simulink model "Sandbox"  (R2023a)
settings: Solver=FixedStepAuto  StartTime=0.0  StopTime=10  FixedStep=0.0001  RelTol=1e-3
values from neighbouring files (symbols this model uses):
  AEP = 0.03    [simulation_setup.m]
  PEP = -0.03    [simulation_setup.m]
  step_height = 0.06    [InitialisationScript.m]    (also in simulation_setup.m)
settings Model: Creator=basti  LastModifiedBy=basti
settings SolverCC: ZeroCrossControl=EnableAll  EnableFixedStepZeroCrossing=on
settings ExplorerConfigSet: InternalSimMechanicsExplorerSettings="<ExplorerConfiguration><canonicalview>planar_xy</canonicalview><AnimationSetting><BasePlaybackSpeed>1.0</BasePlaybackSpeed><PlaybackSpeedFactor>1.0</PlaybackSpeedFactor></AnimationSetting><TilePanel><TileInfo><Tiles Columns=\"1\" Count=\"1\" Rows=\"1\"><Column Weight=\"1\"/><Row Weight=\"1\"/><Tile Height=\"1\" Width=\"1\" X=\"0\" Y=\"0\"/></Tiles></TileInfo><SceneInfo><SceneViewer><BGColor><R>0.800000011920928955</R><G>0.800000011920928955</G><B>0.800000011920928955</B></BGColor><Camera><DoPerspective>off</DoPerspective><Position><X>166.088793964076217</X><Y>-65.4585895917369385</Y><Z>6.56230393982627103</Z></Position><Center><X>0.420963900477701602</X><Y>-0.147668832830340768</Y><Z>0.227388390891763464</Z></Center><Up><X>-0.0260738065319616186</X><Y>0.030778444548253292</Y><Z>0.999186090757934631</Z></Up><ViewLimDist>1</ViewLimDist><YLim>0.165421804575422993</YLim><XLim>0.319699403368922774</XLim></Camera></SceneViewer></SceneInfo></TilePanel><MechEditorPanel><Cameras/><GfxPanelCameraMap/><VideoCreator><PlaybackSpeedRatio>1.0</PlaybackSpeedRatio><FrameRate>30</FrameRate><VideoFormat>Motion JPEG AVI</VideoFormat><FrameSize>auto</FrameSize></VideoCreator></MechEditorPanel></ExplorerConfiguration>"

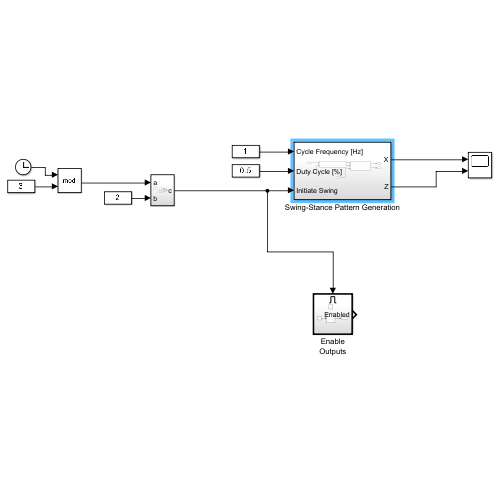
[thumbnail: Simulink's stored preview of the top-level diagram]
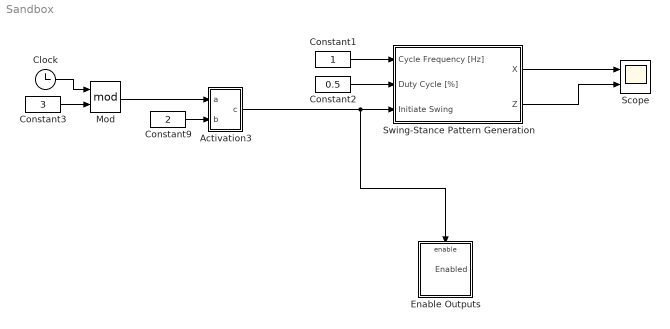
== system Sandbox ==
  Activation3 : Subsystem
  Clock : Clock
  Constant1 : Constant
  Constant2 : Constant  Value=0.5
  Constant3 : Constant  Value=3
  Constant9 : Constant  Value=2
  Enable Outputs : Subsystem  TreatAsAtomicUnit=on
  Mod : Math  Operator=mod
  Scope : Scope  NumInputPorts=2
  Swing-Stance Pattern Generation : Subsystem
  wires:
  Constant9/1 -> Activation3/2(b)
  Swing-Stance Pattern Generation/1(X) -> Scope/1
  Swing-Stance Pattern Generation/2(Z) -> Scope/2
  Activation3/1(c) -> Swing-Stance Pattern Generation/3(Initiate Swing), Enable Outputs/Enable
  Constant2/1 -> Swing-Stance Pattern Generation/2(Duty Cycle [%])
  Constant1/1 -> Swing-Stance Pattern Generation/1(Cycle Frequency [Hz])
  Clock/1 -> Mod/1
  Mod/1 -> Activation3/1(a)
  Constant3/1 -> Mod/2

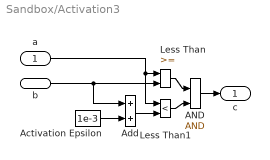
== system Sandbox/Activation3 ==
  a : Inport
  b : Inport  Port=2
  AND : Logic  IconShape=distinctive  AllPortsSameDT=off  OutDataTypeStr=boolean
  Activation Epsilon : Constant  Value=1e-3
  Add : Sum
  Less Than : RelationalOperator  OutDataTypeStr=boolean  RndMeth=Simplest  InputSameDT=off
  Less Than1 : RelationalOperator  Operator=<  OutDataTypeStr=boolean  RndMeth=Simplest  InputSameDT=off
  c : Outport
  wires:
  a/1 -> Less Than1/1, Less Than/1
  Less Than/1 -> AND/1
  Less Than1/1 -> AND/2
  Add/1 -> Less Than1/2
  b/1 -> Add/1, Less Than/2
  AND/1 -> c/1
  Activation Epsilon/1 -> Add/2

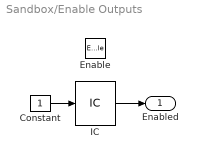
== system Sandbox/Enable Outputs ==
  Enable : EnablePort
  Constant : Constant
  IC : InitialCondition  Value=0
  Enabled : Outport  InitialOutput=0
  wires:
  Constant/1 -> IC/1
  IC/1 -> Enabled/1

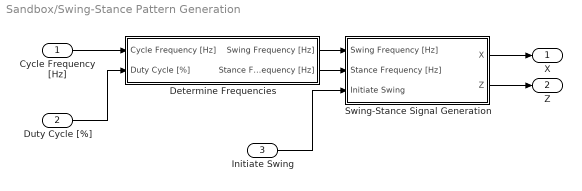
== system Sandbox/Swing-Stance Pattern Generation ==
  Cycle Frequency [Hz] : Inport
  Duty Cycle [%] : Inport  Port=2
  Initiate Swing : Inport  Port=3
  Determine Frequencies : Subsystem
  Swing-Stance Signal Generation : Subsystem
  X : Outport
  Z : Outport  Port=2
  wires:
  Swing-Stance Signal Generation/1(X) -> X/1
  Cycle Frequency [Hz]/1 -> Determine Frequencies/1(Cycle Frequency [Hz])
  Determine Frequencies/1(Swing Frequency [Hz]) -> Swing-Stance Signal Generation/1(Swing Frequency [Hz])
  Initiate Swing/1 -> Swing-Stance Signal Generation/3(Initiate Swing)
  Duty Cycle [%]/1 -> Determine Frequencies/2(Duty Cycle [%])
  Determine Frequencies/2(Stance Frequency [Hz]) -> Swing-Stance Signal Generation/2(Stance Frequency [Hz])
  Swing-Stance Signal Generation/2(Z) -> Z/1

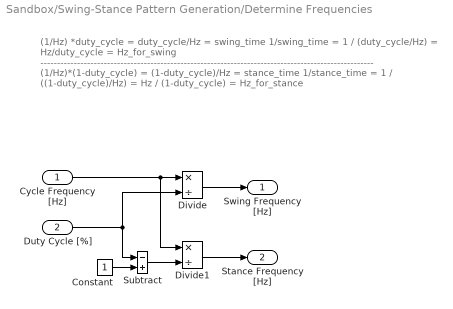
== system Sandbox/Swing-Stance Pattern Generation/Determine Frequencies ==
  note: (1/Hz) *duty_cycle = duty_cycle/Hz = swing_time
      |
      | 1/swing_time = 1 / (duty_cycle/Hz) = Hz/duty_cycle = Hz_for_swing
      | ----------------------------------------------------------------------------------------------------
      | (1/Hz)*(1-duty_cycle) = (1-duty_cycle)/Hz = stance_time
      |
      | 1/stance_time = 1 / ((1-duty_cycle)/Hz) = Hz / (1-duty_cycle) = Hz_for_stance
  Cycle Frequency [Hz] : Inport
  Duty Cycle [%] : Inport  Port=2
  Constant : Constant
  Divide : Product  Inputs=*/
  Divide1 : Product  Inputs=*/
  Subtract : Sum  Inputs=-+
  Swing Frequency [Hz] : Outport
  Stance Frequency [Hz] : Outport  Port=2
  wires:
  Constant/1 -> Subtract/2
  Subtract/1 -> Divide1/2
  Divide1/1 -> Stance Frequency [Hz]/1
  Cycle Frequency [Hz]/1 -> Divide/1, Divide1/1
  Duty Cycle [%]/1 -> Divide/2, Subtract/1
  Divide/1 -> Swing Frequency [Hz]/1

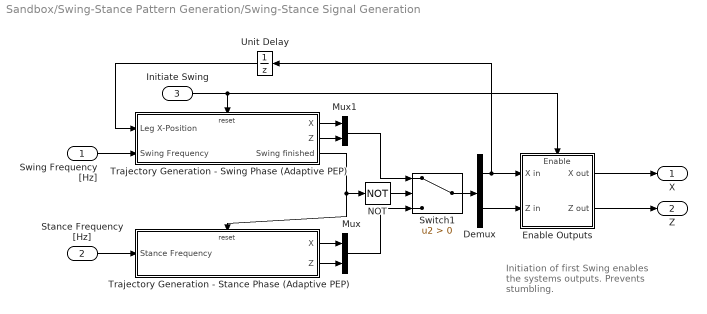
== system Sandbox/Swing-Stance Pattern Generation/Swing-Stance Signal Generation ==
  note: Initiation of first Swing
      | enables the systems outputs.
      | Prevents stumbling.
  Swing Frequency [Hz] : Inport
  Stance Frequency [Hz] : Inport  Port=2
  Initiate Swing : Inport  Port=3
  Demux : Demux  Outputs=2
  Enable Outputs : Subsystem  TreatAsAtomicUnit=on
      settings: PortSchema="{\"entries\":[{\"content\":{\"sides\":[{\"content\":{\"connectorIds\":[\"In1\",\"In2\"]},\"type\":\"ConnectorPlacement.EquallySpacedRectSide\",\"uuid\":\"87b33ceb-5119-42f0-ab9e-44a74532733d\"},{\"content\":{\"connectorIds\":[\"Out1\",\"Out2\"],\"side\":\"RIGHT\"},\"type\":\"ConnectorPlacement.EquallySpacedRectSide\",\"uuid\":\"2748c539-b9f3-4627-a92c-05139a6ac450\"},{\"content\":{\"connectorIds\":[\"In3\"],\"side\":\"TOP\"},\"type\":\"ConnectorPlacement.EquallySpacedRectSide\",\"uuid\":\"98271061-2ac6-4173-8399-340c777b7c0e\"}]},\"type\":\"ConnectorPlacement.EquallySpacedConnector\",\"uuid\":\"a1ce645b-bfd3-4385-aaad-491949d96666\"}],\"packageUris\":[\"http://schema.mathworks.com/mf0/Connector/R2020b\"],\"version\":\"1.0\"}"
  Mux : Mux  Inputs=2
  Mux1 : Mux  Inputs=2
  NOT : Logic  Operator=NOT  IconShape=distinctive  AllPortsSameDT=off  OutDataTypeStr=boolean
  Switch1 : Switch  Criteria=u2 > Threshold  SaturateOnIntegerOverflow=off  InputSameDT=off
  Trajectory Generation - Stance Phase (Adaptive PEP) : Subsystem  TreatAsAtomicUnit=on
  Trajectory Generation - Swing Phase (Adaptive PEP) : Subsystem  TreatAsAtomicUnit=on
  Unit Delay : UnitDelay  SampleTime=-1  HasFrameUpgradeWarning=on
  X : Outport
  Z : Outport  Port=2
  wires:
  Enable Outputs/1(X out) -> X/1
  Enable Outputs/2(Z out) -> Z/1
  Switch1/1 -> Demux/1
  Demux/1 -> Enable Outputs/1(X in), Unit Delay/1
  Unit Delay/1 -> Trajectory Generation - Swing Phase (Adaptive PEP)/1(Leg X-Position)
  Stance Frequency [Hz]/1 -> Trajectory Generation - Stance Phase (Adaptive PEP)/1(Stance Frequency)
  Trajectory Generation - Stance Phase (Adaptive PEP)/2(Z) -> Mux/2
  Trajectory Generation - Swing Phase (Adaptive PEP)/2(Z) -> Mux1/2
  Trajectory Generation - Stance Phase (Adaptive PEP)/1(X) -> Mux/1
  Mux1/1 -> Switch1/1
  Trajectory Generation - Swing Phase (Adaptive PEP)/1(X) -> Mux1/1
  Demux/2 -> Enable Outputs/2(Z in)
  Mux/1 -> Switch1/3
  Initiate Swing/1 -> Enable Outputs/3(Enable), Trajectory Generation - Swing Phase (Adaptive PEP)/Reset
  NOT/1 -> Switch1/2
  Trajectory Generation - Swing Phase (Adaptive PEP)/3(Swing finished) -> NOT/1, Trajectory Generation - Stance Phase (Adaptive PEP)/Reset
  Swing Frequency [Hz]/1 -> Trajectory Generation - Swing Phase (Adaptive PEP)/2(Swing Frequency)

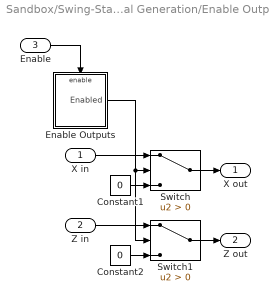
== system Sandbox/Swing-Stance Pattern Generation/Swing-Stance Signal Generation/Enable Outputs ==
  X in : Inport
  Z in : Inport  Port=2
  Enable : Inport  Port=3
  Constant1 : Constant  Value=0
  Constant2 : Constant  Value=0
  Enable Outputs : Subsystem  TreatAsAtomicUnit=on
  Switch : Switch  Criteria=u2 > Threshold  SaturateOnIntegerOverflow=off  InputSameDT=off
  Switch1 : Switch  Criteria=u2 > Threshold  SaturateOnIntegerOverflow=off  InputSameDT=off
  X out : Outport  InitialOutput=0
  Z out : Outport  Port=2  InitialOutput=0
  wires:
  Switch1/1 -> Z out/1
  Z in/1 -> Switch1/1
  Constant2/1 -> Switch1/3
  Constant1/1 -> Switch/3
  X in/1 -> Switch/1
  Switch/1 -> X out/1
  Enable/1 -> Enable Outputs/Enable
  Enable Outputs/1(Enabled) -> Switch1/2, Switch/2

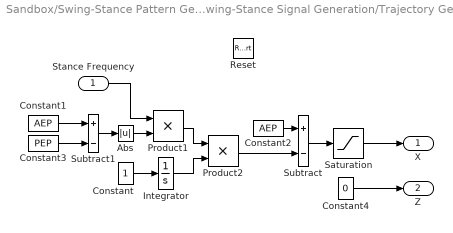
== system Sandbox/Swing-Stance Pattern Generation/Swing-Stance Signal Generation/Trajectory Generation - Stance Phase (Adaptive PEP) ==
  Stance Frequency : Inport
  Reset : ResetPort  DisableCoverage=on
  Abs : Abs  SaturateOnIntegerOverflow=off
  Constant : Constant
  Constant1 : Constant  Value=AEP
  Constant2 : Constant  Value=AEP
  Constant3 : Constant  Value=PEP
  Constant4 : Constant  Value=0
  Integrator : Integrator
  Product1 : Product
  Product2 : Product
  Saturation : Saturate  UpperLimit=AEP  LowerLimit=PEP
  Subtract : Sum  Inputs=+-
  Subtract1 : Sum  Inputs=+-
  X : Outport
  Z : Outport  Port=2
  wires:
  Constant4/1 -> Z/1
  Saturation/1 -> X/1
  Product1/1 -> Product2/1
  Abs/1 -> Product1/2
  Subtract1/1 -> Abs/1
  Constant3/1 -> Subtract1/2
  Constant1/1 -> Subtract1/1
  Stance Frequency/1 -> Product1/1
  Integrator/1 -> Product2/2
  Product2/1 -> Subtract/2
  Subtract/1 -> Saturation/1
  Constant2/1 -> Subtract/1
  Constant/1 -> Integrator/1

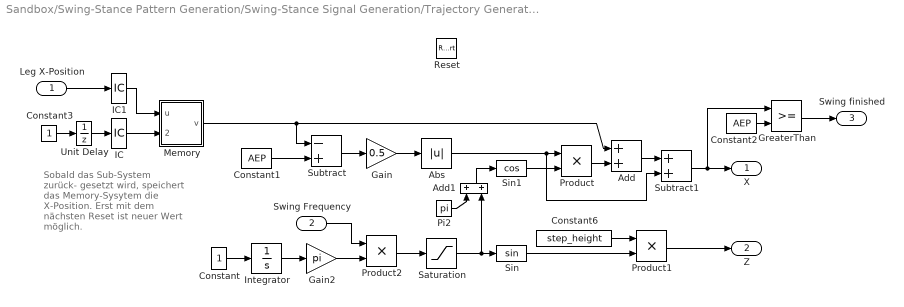
== system Sandbox/Swing-Stance Pattern Generation/Swing-Stance Signal Generation/Trajectory Generation - Swing Phase (Adaptive PEP) ==
  note: Sobald das Sub-System zurück-
      | gesetzt wird, speichert das
      | Memory-Sysytem die X-Position.
      | Erst mit dem nächsten Reset ist
      | neuer Wert möglich.
  Leg X-Position : Inport
  Swing Frequency : Inport  Port=2
  Reset : ResetPort  DisableCoverage=on
  Abs : Abs  SaturateOnIntegerOverflow=off
  Add : Sum
  Add1 : Sum
  Constant : Constant
  Constant1 : Constant  Value=AEP
  Constant2 : Constant  Value=AEP
  Constant3 : Constant
  Constant6 : Constant  Value=step_height
  Gain : Gain  Gain=0.5
  Gain2 : Gain  Gain=pi
  GreaterThan : RelationalOperator  OutDataTypeStr=boolean  RndMeth=Simplest  InputSameDT=off
  IC : InitialCondition  Value=0
  IC1 : InitialCondition  Value=0
  Integrator : Integrator
  Memory : Subsystem
  Pi2 : Constant  Value=pi  OutDataTypeStr=Inherit: Inherit via back propagation
  Product : Product
  Product1 : Product
  Product2 : Product
  Saturation : Saturate  UpperLimit=pi  LowerLimit=0
  Sin : Trigonometry
  Sin1 : Trigonometry  Operator=cos
  Subtract : Sum  Inputs=-+
  Subtract1 : Sum
  Unit Delay : UnitDelay  SampleTime=-1  HasFrameUpgradeWarning=on
  X : Outport
  Z : Outport  Port=2
  Swing finished : Outport  Port=3
  wires:
  IC1/1 -> Memory/1(u)
  IC/1 -> Memory/2(Hold)
  Constant3/1 -> Unit Delay/1
  Unit Delay/1 -> IC/1
  Leg X-Position/1 -> IC1/1
  Swing Frequency/1 -> Product2/1
  Product2/1 -> Saturation/1
  Gain2/1 -> Product2/2
  Constant2/1 -> GreaterThan/2
  GreaterThan/1 -> Swing finished/1
  Constant/1 -> Integrator/1
  Integrator/1 -> Gain2/1
  Subtract1/1 -> GreaterThan/1, X/1
  Sin/1 -> Product1/2
  Gain/1 -> Abs/1
  Constant6/1 -> Product1/1
  Saturation/1 -> Sin/1, Add1/2
  Pi2/1 -> Add1/1
  Memory/1(v) -> Subtract/1, Add/1
  Product1/1 -> Z/1
  Constant1/1 -> Subtract/2
  Sin1/1 -> Product/2
  Add1/1 -> Sin1/1
  Add/1 -> Subtract1/1
  Subtract/1 -> Gain/1
  Abs/1 -> Product/1, Subtract1/2
  Product/1 -> Add/2

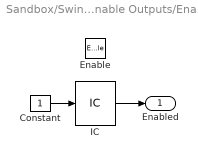
== system Sandbox/Swing-Stance Pattern Generation/Swing-Stance Signal Generation/Enable Outputs/Enable Outputs ==
  Enable : EnablePort
  Constant : Constant
  IC : InitialCondition  Value=0
  Enabled : Outport  InitialOutput=0
  wires:
  Constant/1 -> IC/1
  IC/1 -> Enabled/1

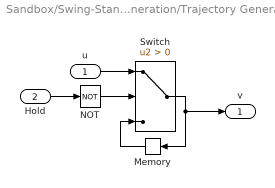
== system Sandbox/Swing-Stance Pattern Generation/Swing-Stance Signal Generation/Trajectory Generation - Swing Phase (Adaptive PEP)/Memory ==
  u : Inport
  Hold : Inport  Port=2
  Memory : Memory
  NOT : Logic  Operator=NOT  IconShape=distinctive  AllPortsSameDT=off  OutDataTypeStr=boolean
  Switch : Switch  Criteria=u2 > Threshold  SaturateOnIntegerOverflow=off  InputSameDT=off
  v : Outport
  wires:
  Memory/1 -> Switch/3
  u/1 -> Switch/1
  NOT/1 -> Switch/2
  Hold/1 -> NOT/1
  Switch/1 -> Memory/1, v/1
